simulink subsystem "Day1_Scenario_3_4"  (R2024a)
settings: Solver=VariableStepAuto  StartTime=0.0  StopTime=10.0  RelTol=1e-3
libraries: CarMaker4SL x3
settings Model: Creator=junhyung.cha  LastModifiedBy=User

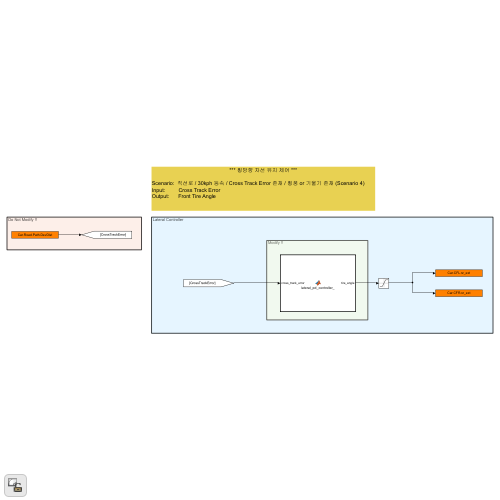
[thumbnail: Simulink's stored preview of the top-level diagram]
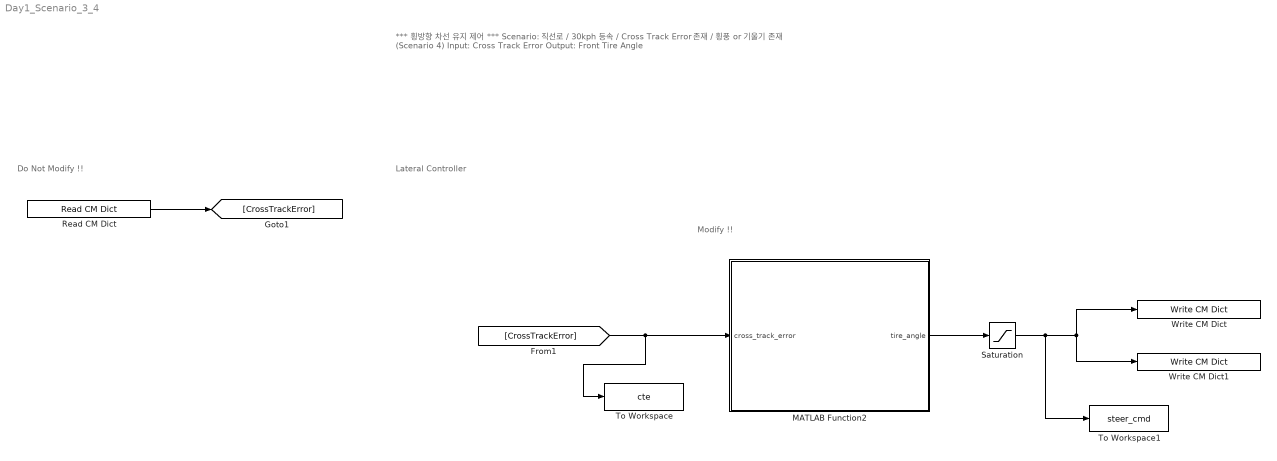
== system Day1_Scenario_3_4 ==
  note: Do Not Modify !!
  note: Modify !!
  note: Lateral Controller
  note: *** 횡방향 차선 유지 제어 ***
      |
      | Scenario: 직선로 / 30kph 등속 / Cross Track Error 존재 / 횡풍 or 기울기 존재 (Scenario 4)
      | Input: Cross Track Error
      | Output: Front Tire Angle
  MATLAB Function2 : MATLAB Function  TreatAsAtomicUnit=on
  Read CM Dict : CarMaker4SL/Read CM Dict  xname=Car.Road.Path.DevDist  xsync=off  xstime=Inherited
  Saturation : Saturate  UpperLimit=2  LowerLimit=-2
  To Workspace : ToWorkspace  VariableName=cte  SaveFormat=Timeseries  SampleTime=-1
  To Workspace1 : ToWorkspace  VariableName=steer_cmd  SaveFormat=Timeseries  SampleTime=-1
  Write CM Dict : CarMaker4SL/Write CM Dict  xname=Car.CFL.rz_ext  xsync=off
  Write CM Dict1 : CarMaker4SL/Write CM Dict  xname=Car.CFR.rz_ext  xsync=off
  wires:
  Read CM Dict/1 -> [CrossTrackError]
  MATLAB Function2/1(tire_angle) -> Saturation/1
  [CrossTrackError] -> MATLAB Function2/1(cross_track_error), To Workspace/1
  Saturation/1 -> Write CM Dict/1, Write CM Dict1/1, To Workspace1/1

== matlab function Day1_Scenario_3_4/MATLAB Function2 ==
  settings: updateMethod=DISCRETE  sampleTime=0.05
  data: cross_track_error input; tire_angle output
function tire_angle = lateral_pd_controller_(cross_track_error)
  persistent prev_e int_e initialized

  dt = 0.001;
  Kp = 0.09;
  Kd = 0.002;
  Ki = 0.03;

  dir = -1;

  e = cross_track_error;

  if isempty(initialized)
      prev_e = e;
      int_e = 0;
      initialized = true;
  end

  d_e = (e - prev_e) / dt;

  int_e = int_e + e * dt;

  tire_angle = dir * (Kp * e + Kd * d_e + Ki * int_e);


  prev_e = e;
end
